simulink model "Solarzelle_Simulink"  (R2022b)
settings: Solver=VariableStepAuto  StartTime=0.0  StopTime=100  RelTol=1e-3
settings Model: Creator=chris  LastModifiedBy=chris
settings ModelReferenceCC: EnableRefExpFcnMdlSchedulingChecks=on

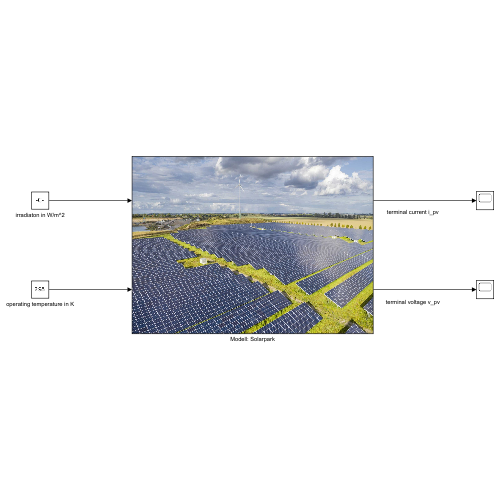
[thumbnail: Simulink's stored preview of the top-level diagram]
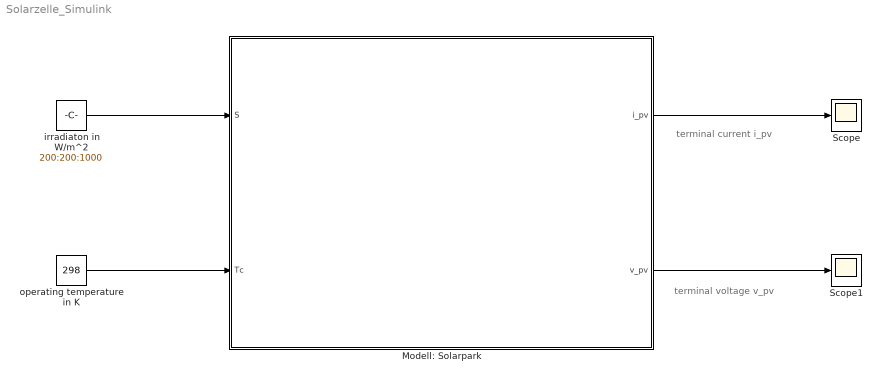
== system Solarzelle_Simulink ==
  note: terminal voltage v_pv
  note: terminal current i_pv
  Modell: Solarpark : Subsystem
      mask Display: image('$imagefile'); % Use "Edit Image" on toolstrip to change.
  Scope : Scope
  Scope1 : Scope
  irradiaton in W/m^2 : Constant  Value=200:200:1000
  operating temperature in K : Constant  Value=298
  wires:
  irradiaton in W/m^2/1 -> Modell: Solarpark/1(S)
  Modell: Solarpark/1(i_pv) -> Scope/1
  Modell: Solarpark/2(v_pv) -> Scope1/1
  operating temperature in K/1 -> Modell: Solarpark/2(Tc)

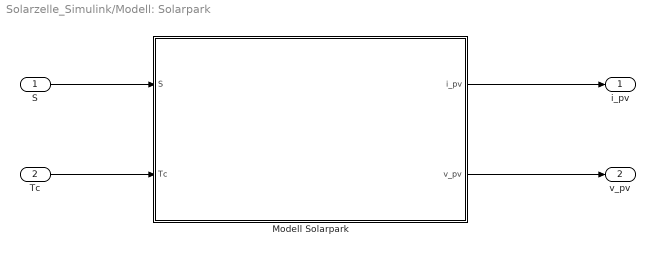
== system Solarzelle_Simulink/Modell: Solarpark ==
  S : Inport
  Tc : Inport  Port=2
  Modell Solarpark : MATLAB Function  TreatAsAtomicUnit=on
  i_pv : Outport
  v_pv : Outport  Port=2
  wires:
  Modell Solarpark/1(i_pv) -> i_pv/1
  S/1 -> Modell Solarpark/1(S)
  Tc/1 -> Modell Solarpark/2(Tc)
  Modell Solarpark/2(v_pv) -> v_pv/1

== matlab function Solarzelle_Simulink/Modell: Solarpark/Modell Solarpark ==
  data: S input; i_pv output; param parameter; Tc input; v_pv output
function [i_pv, v_pv] = fcn(S, param, Tc) 

% 1. Gleichung: Photodiodenstrom
i_ph = S/param.S_STC * param.iph_SC_STC *(1 + param.alpha_T * (Tc-param.Tc_STC)); 

%Berechnung der Leerlaufspannung für i_s
v_OC = param.v_OC_STC * (1 + param.beta_T * (Tc-param.Tc_STC));

% 2. Gleichung: Irgendwas Strom
i_s = (i_ph - (v_OC/param.Rh))/(exp(v_OC/(param.An * param.vT_STC))-1);

% 3. Gleichung: Bypass-Diodenstrom
i_d = i_s * (exp(param.v_pv_z/(param.An*param.vT_STC))-1);

% Resultierender Strom aller paralellgeschalteter Solarzellen;
i_pv = param.Np * i_ph - param.Np * i_d - (param.Np/param.Ns) * (param.v_pv_z/param.Rh);

%Resultierende Spannungswerte aller in reihegeschalteter Solarzellen
v_pv = param.Ns * param.v_pv_z;

end
